simulink model "Haptic feedbck system"  (R2024b)
settings: Solver=ode4  StartTime=0.0  StopTime=inf  FixedStep=0.001  RelTol=1e-3  EnableMultiTasking=on
undefined symbols (not defined in the file): _, cablePTstudyZF, data, date, DiscIntNeverNeededParam, FETau, HIL, i2tTimeLim, iCmd2Volt, iCmdLim, iCmdSat, iCont, iMeasLim, iMeasServoConv, iPeak, iSign, kDposStudyPC, kDstudyZF, kPposStudyPC, kPstudyZF, kS, magnitude, maxTorque, motEncCnts2Rad, motEncSign, motKt, motNegFfTauStudyPC, motPosFfTauStudyPC, motPulleyRad, pulseGuiPeriod, pulseGuiPulseWidth, qc_get_step_size, signals, sprEncCnts2Rad, sprEncSign, tauDzStudyZF, tauJlim, tauMlim, tauNoMvtStudyZF, test_1_robot_torque_, time, tS, Visualization, xJdotLim, xJlimNeg, xJlimPos, xMdotLim, xMlimNeg, xMlimPos
libraries: quarc_library x26, simulink x13, simulink_extras x2
(part 2 of 3)

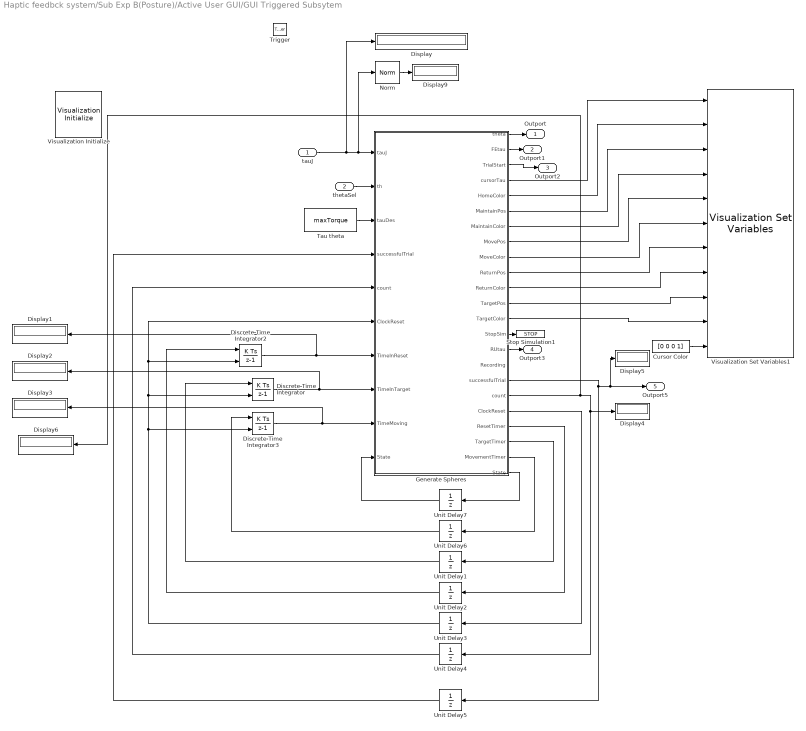
== system Haptic feedbck system/Sub Exp B(Posture)/Active User GUI/GUI Triggered Subsytem ==
  tauJ : Inport
  thetaSel : Inport  Port=2
  Trigger : TriggerPort  VariantControl=(inherit)
  Cursor Color : Constant  Value=[0 0 0 1]  VectorParams1D=off
  Discrete-Time Integrator : DiscreteIntegrator  ExternalReset=rising  SampleTime=-1  OutDataTypeStr=double  ICPrevOutput=DiscIntNeverNeededParam  ICPrevScaledInput=DiscIntNeverNeededParam
  Discrete-Time Integrator2 : DiscreteIntegrator  ExternalReset=rising  SampleTime=-1  OutDataTypeStr=double  ICPrevOutput=DiscIntNeverNeededParam  ICPrevScaledInput=DiscIntNeverNeededParam
  Discrete-Time Integrator3 : DiscreteIntegrator  ExternalReset=rising  SampleTime=-1  OutDataTypeStr=double  ICPrevOutput=DiscIntNeverNeededParam  ICPrevScaledInput=DiscIntNeverNeededParam
  Display{,1..6,9} (8 alike) : Display
  Generate Spheres : MATLAB Function  TreatAsAtomicUnit=on
  Norm : quarc_library/Math Operations/Vectors/Norm
      settings: SourceProductName=QUARC Targets
  Stop Simulation1 : Stop
  Tau theta : Constant  Value=maxTorque  SampleTime=-1
  Unit Delay{1..6} (6 alike) : UnitDelay  SampleTime=-1  HasFrameUpgradeWarning=on
  Unit Delay7 : UnitDelay  InitialCondition=1  SampleTime=-1  StateName=State  HasFrameUpgradeWarning=on
  Visualization Initialize : quarc_library/User Interface/Visualization/Visualization Initialize  object_name=Visualization-1  scene_file=untitled.xml  uri=shmem://%m:1?private=visual  server_send_size=1000000  server_receive_size=1000  derive_from_server=on  client_send_size=1000  client_receive_size=1000000  variables=[ 20 24 34 40 44 50 54 60 64 70 74 ]  initial_values=single([ 0 0 0 1 1 1 1 1 1 1 1 -0.01 0 0 0 0 0 1 0 0 1 0 1 0 1 0 0 0 1 1 1 1 0 0 0 1 1 1 1 ])  open_on_start=on  close_on_stop=off
      settings: AttributesFormatString=%<object_name>  SourceProductName=QUARC Targets
  Visualization Set Variables1 : quarc_library/User Interface/Visualization/Visualization Set Variables  object_name=Visualization-1  offset=[ 11 7 32 35 0 3 25 28 18 21 14 ]  data_type=[ 0 0 0 0 0 0 0 0 0 0 0 ]  length=[ 3 4 3 4 3 4 3 4 3 4 4 ]  sample_time=visualization_get_frame_period  actor_name={'actor.cursor/Position';'actor.home/Diffuse Color';'actor.maintain/Position';'actor.maintain/Diffuse Color';'actor.move/Position';'actor.move/Diffuse Color';'actor.return/Position';'actor.return/Diffuse Color';'actor.target/Position';'actor.target/Diffuse Color';'actor.cursor/Diffuse Color'}
      settings: AttributesFormatString=(%<object_name>)  SourceProductName=QUARC Targets
  Outport : Outport
  Outport1 : Outport  Port=2
  Outport2 : Outport  Port=3
  Outport3 : Outport  Port=4
  Outport5 : Outport  Port=5
  wires:
  thetaSel/1 -> Generate Spheres/2(th)
  Tau theta/1 -> Generate Spheres/3(tauDes)
  tauJ/1 -> Display/1, Norm/1, Generate Spheres/1(tauJ)
  Generate Spheres/19(ClockReset) -> Unit Delay3/1
  Generate Spheres/4(cursorTau) -> Visualization Set Variables1/1
  Generate Spheres/21(TargetTimer) -> Unit Delay1/1
  Unit Delay4/1 -> Generate Spheres/5("count ")
  Generate Spheres/17(successfulTrial) -> Display5/1, Outport5/1, Unit Delay5/1
  Unit Delay5/1 -> Generate Spheres/4("successfulTrial ")
  Unit Delay3/1 -> Generate Spheres/6("ClockReset "), Discrete-Time Integrator2/2, Discrete-Time Integrator/2, Discrete-Time Integrator3/2
  Norm/1 -> Display9/1
  Generate Spheres/20(ResetTimer) -> Unit Delay2/1
  Discrete-Time Integrator3/1 -> Display3/1, Generate Spheres/9(TimeMoving)
  Generate Spheres/22(MovementTimer) -> Unit Delay6/1
  Unit Delay2/1 -> Discrete-Time Integrator2/1
  Discrete-Time Integrator2/1 -> Display1/1, Generate Spheres/7(TimeInReset)
  Unit Delay1/1 -> Discrete-Time Integrator/1
  Unit Delay6/1 -> Discrete-Time Integrator3/1
  Discrete-Time Integrator/1 -> Display2/1, Generate Spheres/8(TimeInTarget)
  Generate Spheres/23(State) -> Unit Delay7/1
  Unit Delay7/1 -> Generate Spheres/10("State ")
  Generate Spheres/5(HomeColor) -> Visualization Set Variables1/2
  Generate Spheres/6(MaintainPos) -> Visualization Set Variables1/3
  Generate Spheres/7(MaintainColor) -> Visualization Set Variables1/4
  Generate Spheres/8(MovePos) -> Visualization Set Variables1/5
  Generate Spheres/9(MoveColor) -> Visualization Set Variables1/6
  Generate Spheres/10(ReturnPos) -> Visualization Set Variables1/7
  Generate Spheres/11(ReturnColor) -> Visualization Set Variables1/8
  Generate Spheres/12(TargetPos) -> Visualization Set Variables1/9
  Generate Spheres/13(TargetColor) -> Visualization Set Variables1/10
  Cursor Color/1 -> Visualization Set Variables1/11
  Generate Spheres/1(theta) -> Outport/1
  Generate Spheres/2(FEtau) -> Outport1/1
  Generate Spheres/3(TrialStart) -> Outport2/1
  Generate Spheres/15(RUtau) -> Outport3/1
  Generate Spheres/14(StopSim) -> Stop Simulation1/1
  Generate Spheres/18(count) -> Display6/1, Display4/1, Unit Delay4/1

== system Haptic feedbck system/Sub Exp B(Posture)/Active UserData Recording/Enabled Subsystem1 ==
  In1 : Inport
  Enable : EnablePort
  To Host File : quarc_library/Sinks/To Host/To Host File  source=Specify via dialog (do not evaluate)  file_name=Main_study_p3_C2_F_R1  variable_name=data  decimation=1  sample_time=-1  file_format=CSV-file  options=Include header only  append=off  final_file_name=Main_study_p3_C2_F_R1.csv  bitrate=2000000
  wires:
  In1/1 -> To Host File/1

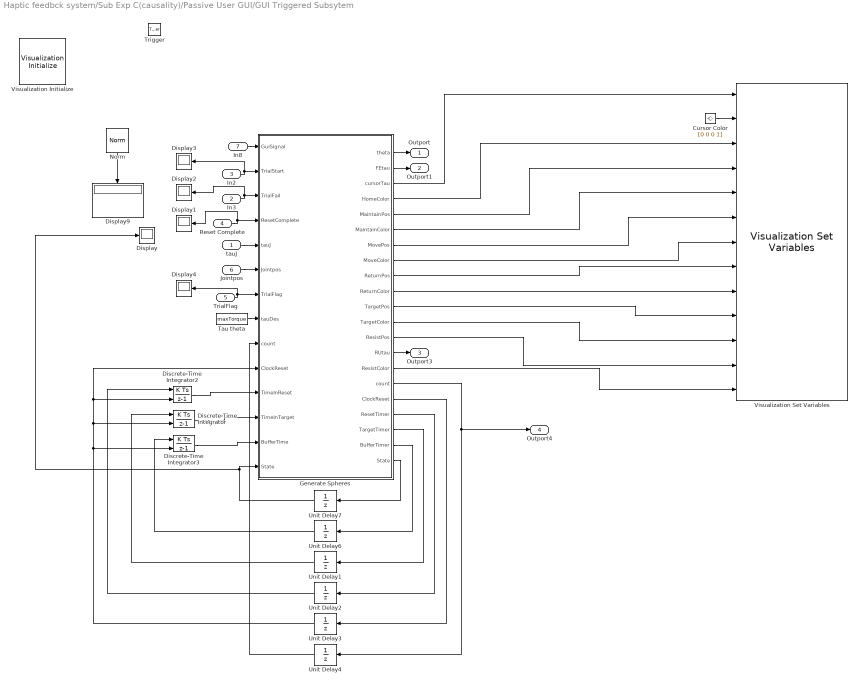
== system Haptic feedbck system/Sub Exp C(causality)/Passive User GUI/GUI Triggered Subsytem ==
  tauJ : Inport
  In3 : Inport  Port=2
  In2 : Inport  Port=3
  Reset Complete : Inport  Port=4
  TrialFlag : Inport  Port=5
  Jointpos : Inport  Port=6
  In8 : Inport  Port=7
  Trigger : TriggerPort  VariantControl=(inherit)
  Cursor Color : Constant  Value=[0 0 0 1]  VectorParams1D=off
  Discrete-Time Integrator : DiscreteIntegrator  ExternalReset=rising  SampleTime=-1  OutDataTypeStr=double  ICPrevOutput=DiscIntNeverNeededParam  ICPrevScaledInput=DiscIntNeverNeededParam
  Discrete-Time Integrator2 : DiscreteIntegrator  ExternalReset=rising  SampleTime=-1  OutDataTypeStr=double  ICPrevOutput=DiscIntNeverNeededParam  ICPrevScaledInput=DiscIntNeverNeededParam
  Discrete-Time Integrator3 : DiscreteIntegrator  ExternalReset=rising  SampleTime=-1  OutDataTypeStr=double  ICPrevOutput=DiscIntNeverNeededParam  ICPrevScaledInput=DiscIntNeverNeededParam
  Display{,1..4,9} (6 alike) : Display
  Generate Spheres : MATLAB Function  TreatAsAtomicUnit=on
  Norm : quarc_library/Math Operations/Vectors/Norm
      settings: SourceProductName=QUARC Targets
  Tau theta : Constant  Value=maxTorque  SampleTime=-1
  Unit Delay{1..4,6} (5 alike) : UnitDelay  SampleTime=-1  HasFrameUpgradeWarning=on
  Unit Delay7 : UnitDelay  SampleTime=-1  StateName=State  HasFrameUpgradeWarning=on
  Visualization Initialize : quarc_library/User Interface/Visualization/Visualization Initialize  object_name=Visualization-1  scene_file=..\exp files\untitled.xml  uri=shmem://%m:1?private=visual  server_send_size=1000000  server_receive_size=1000  derive_from_server=on  client_send_size=1000  client_receive_size=1000000  variables=[ 20 24 30 34 44 50 54 60 64 70 74 80 84 ]  initial_values=single([ -0.01 0 0 0 0 0 1 0 0 0 1 1 1 1 1 1 1 1 0 0 0 1 1 1 1 0 0 0 1 1 1 1 0 0 0 1 1 1 1 0 0 0 1 1 1 1 ])  open_on_start=on  close_on_stop=off
      settings: AttributesFormatString=%<object_name>  SourceProductName=QUARC Targets
  Visualization Set Variables : quarc_library/User Interface/Visualization/Visualization Set Variables  object_name=Visualization-1  offset=[ 0 3 14 25 28 18 21 32 35 7 10 39 42 ]  data_type=[ 0 0 0 0 0 0 0 0 0 0 0 0 0 ]  length=[ 3 4 4 3 4 3 4 3 4 3 4 3 4 ]  sample_time=visualization_get_frame_period  actor_name={'actor.cursor/Position';'actor.cursor/Diffuse Color';'actor.home/Diffuse Color';'actor.maintain/Position';'actor.maintain/Diffuse Color';'actor.move/Position';'actor.move/Diffuse Color';'actor.return/Position';'actor.return/Diffuse Color';'actor.target/Position';'actor.target/Diffuse Color';'actor.resist/Position';'actor.resist/Diffuse Color'}
      settings: AttributesFormatString=(%<object_name>)  SourceProductName=QUARC Targets
  Outport : Outport
  Outport1 : Outport  Port=2
  Outport3 : Outport  Port=3
  Outport4 : Outport  Port=4
  wires:
  Generate Spheres/17(ClockReset) -> Unit Delay3/1
  Generate Spheres/19(TargetTimer) -> Unit Delay1/1
  Unit Delay4/1 -> Generate Spheres/9("count ")
  Unit Delay3/1 -> Generate Spheres/10("ClockReset "), Discrete-Time Integrator2/2, Discrete-Time Integrator/2, Discrete-Time Integrator3/2
  Norm/1 -> Display9/1
  Generate Spheres/18(ResetTimer) -> Unit Delay2/1
  Discrete-Time Integrator3/1 -> Generate Spheres/13(BufferTime)
  Generate Spheres/20(BufferTimer) -> Unit Delay6/1
  Unit Delay2/1 -> Discrete-Time Integrator2/1
  Discrete-Time Integrator2/1 -> Generate Spheres/11(TimeInReset)
  Unit Delay6/1 -> Discrete-Time Integrator3/1
  Discrete-Time Integrator/1 -> Generate Spheres/12(TimeInTarget)
  Generate Spheres/21(State) -> Unit Delay7/1
  Unit Delay7/1 -> Generate Spheres/14("State "), Display/1
  Generate Spheres/1(theta) -> Outport/1
  Generate Spheres/2(FEtau) -> Outport1/1
  Generate Spheres/14(RUtau) -> Outport3/1
  Unit Delay1/1 -> Discrete-Time Integrator/1
  Generate Spheres/3(cursorTau) -> Visualization Set Variables/1
  Cursor Color/1 -> Visualization Set Variables/2
  Generate Spheres/4(HomeColor) -> Visualization Set Variables/3
  Generate Spheres/5(MaintainPos) -> Visualization Set Variables/4
  Generate Spheres/6(MaintainColor) -> Visualization Set Variables/5
  Generate Spheres/7(MovePos) -> Visualization Set Variables/6
  Generate Spheres/8(MoveColor) -> Visualization Set Variables/7
  Generate Spheres/9(ReturnPos) -> Visualization Set Variables/8
  Generate Spheres/10(ReturnColor) -> Visualization Set Variables/9
  Generate Spheres/11(TargetPos) -> Visualization Set Variables/10
  Generate Spheres/12(TargetColor) -> Visualization Set Variables/11
  Generate Spheres/16(count) -> Outport4/1, Unit Delay4/1
  Generate Spheres/13(ResistPos) -> Visualization Set Variables/12
  Generate Spheres/15(ResistColor) -> Visualization Set Variables/13
  tauJ/1 -> Generate Spheres/5(tauJ)
  Jointpos/1 -> Generate Spheres/6(Jointpos)
  TrialFlag/1 -> Display4/1, Generate Spheres/7(TrialFlag)
  Tau theta/1 -> Generate Spheres/8(tauDes)
  Reset Complete/1 -> Generate Spheres/4(ResetComplete), Display1/1
  In3/1 -> Display2/1, Generate Spheres/3(TrialFail)
  In2/1 -> Display3/1, Generate Spheres/2(TrialStart)
  In8/1 -> Generate Spheres/1(GuiSignal)

== system Haptic feedbck system/Sub Exp C(causality)/Passive UserData Recording/Enabled Subsystem1 ==
  In1 : Inport
  Enable : EnablePort
  To Host File : quarc_library/Sinks/To Host/To Host File  source=Specify via dialog (do not evaluate)  file_name=Main_study_p3_C3_R1  variable_name=data  decimation=1  sample_time=-1  file_format=CSV-file  options=Include header only  append=off  final_file_name=Main_study_p3_C3_R1.csv  bitrate=2000000
  wires:
  In1/1 -> To Host File/1

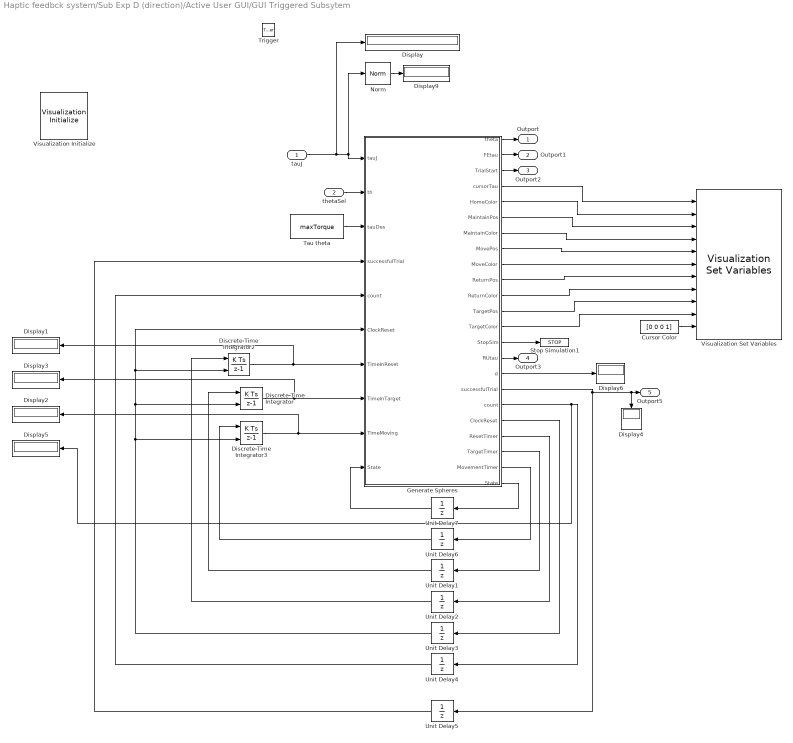
== system Haptic feedbck system/Sub Exp D (direction)/Active User GUI/GUI Triggered Subsytem ==
  tauJ : Inport
  thetaSel : Inport  Port=2
  Trigger : TriggerPort  VariantControl=(inherit)
  Cursor Color : Constant  Value=[0 0 0 1]  VectorParams1D=off
  Discrete-Time Integrator : DiscreteIntegrator  ExternalReset=rising  SampleTime=-1  OutDataTypeStr=double  ICPrevOutput=DiscIntNeverNeededParam  ICPrevScaledInput=DiscIntNeverNeededParam
  Discrete-Time Integrator2 : DiscreteIntegrator  ExternalReset=rising  SampleTime=-1  OutDataTypeStr=double  ICPrevOutput=DiscIntNeverNeededParam  ICPrevScaledInput=DiscIntNeverNeededParam
  Discrete-Time Integrator3 : DiscreteIntegrator  ExternalReset=rising  SampleTime=-1  OutDataTypeStr=double  ICPrevOutput=DiscIntNeverNeededParam  ICPrevScaledInput=DiscIntNeverNeededParam
  Display{,1..6,9} (8 alike) : Display
  Generate Spheres : MATLAB Function  TreatAsAtomicUnit=on
  Norm : quarc_library/Math Operations/Vectors/Norm
      settings: SourceProductName=QUARC Targets
  Stop Simulation1 : Stop
  Tau theta : Constant  Value=maxTorque  SampleTime=-1
  Unit Delay{1..6} (6 alike) : UnitDelay  SampleTime=-1  HasFrameUpgradeWarning=on
  Unit Delay7 : UnitDelay  InitialCondition=1  SampleTime=-1  StateName=State  HasFrameUpgradeWarning=on
  Visualization Initialize : quarc_library/User Interface/Visualization/Visualization Initialize  object_name=Visualization-2  scene_file=untitled.xml  uri=shmem://%m:1?private=visual  server_send_size=1000000  server_receive_size=1000  derive_from_server=on  client_send_size=1000  client_receive_size=1000000  variables=[ 20 24 34 40 44 50 54 60 64 70 74 ]  initial_values=single([ 0 0 0 1 1 1 1 1 1 1 1 -0.01 0 0 0 0 0 1 0 0 1 0 1 0 1 0 0 0 1 1 1 1 0 0 0 1 1 1 1 ])  open_on_start=on  close_on_stop=off
      settings: AttributesFormatString=%<object_name>  SourceProductName=QUARC Targets
  Visualization Set Variables : quarc_library/User Interface/Visualization/Visualization Set Variables  object_name=Visualization-2  offset=[ 11 7 32 35 0 3 25 28 18 21 14 ]  data_type=[ 0 0 0 0 0 0 0 0 0 0 0 ]  length=[ 3 4 3 4 3 4 3 4 3 4 4 ]  sample_time=visualization_get_frame_period  actor_name={'actor.cursor/Position';'actor.home/Diffuse Color';'actor.maintain/Position';'actor.maintain/Diffuse Color';'actor.move/Position';'actor.move/Diffuse Color';'actor.return/Position';'actor.return/Diffuse Color';'actor.target/Position';'actor.target/Diffuse Color';'actor.cursor/Diffuse Color'}
      settings: AttributesFormatString=(%<object_name>)  SourceProductName=QUARC Targets
  Outport : Outport
  Outport1 : Outport  Port=2
  Outport2 : Outport  Port=3
  Outport3 : Outport  Port=4
  Outport5 : Outport  Port=5
  wires:
  thetaSel/1 -> Generate Spheres/2(th)
  Tau theta/1 -> Generate Spheres/3(tauDes)
  tauJ/1 -> Display/1, Norm/1, Generate Spheres/1(tauJ)
  Generate Spheres/19(ClockReset) -> Unit Delay3/1
  Generate Spheres/4(cursorTau) -> Visualization Set Variables/1
  Generate Spheres/21(TargetTimer) -> Unit Delay1/1
  Unit Delay4/1 -> Generate Spheres/5("count ")
  Generate Spheres/17(successfulTrial) -> Display4/1, Outport5/1, Unit Delay5/1
  Unit Delay5/1 -> Generate Spheres/4("successfulTrial ")
  Unit Delay3/1 -> Generate Spheres/6("ClockReset "), Discrete-Time Integrator2/2, Discrete-Time Integrator/2, Discrete-Time Integrator3/2
  Norm/1 -> Display9/1
  Generate Spheres/20(ResetTimer) -> Unit Delay2/1
  Discrete-Time Integrator3/1 -> Display2/1, Generate Spheres/9(TimeMoving)
  Generate Spheres/22(MovementTimer) -> Unit Delay6/1
  Unit Delay2/1 -> Discrete-Time Integrator2/1
  Discrete-Time Integrator2/1 -> Display1/1, Generate Spheres/7(TimeInReset)
  Unit Delay1/1 -> Discrete-Time Integrator/1
  Unit Delay6/1 -> Discrete-Time Integrator3/1
  Discrete-Time Integrator/1 -> Display3/1, Generate Spheres/8(TimeInTarget)
  Generate Spheres/23(State) -> Unit Delay7/1
  Unit Delay7/1 -> Generate Spheres/10("State ")
  Generate Spheres/5(HomeColor) -> Visualization Set Variables/2
  Generate Spheres/6(MaintainPos) -> Visualization Set Variables/3
  Generate Spheres/7(MaintainColor) -> Visualization Set Variables/4
  Generate Spheres/8(MovePos) -> Visualization Set Variables/5
  Generate Spheres/9(MoveColor) -> Visualization Set Variables/6
  Generate Spheres/10(ReturnPos) -> Visualization Set Variables/7
  Generate Spheres/11(ReturnColor) -> Visualization Set Variables/8
  Generate Spheres/12(TargetPos) -> Visualization Set Variables/9
  Generate Spheres/13(TargetColor) -> Visualization Set Variables/10
  Cursor Color/1 -> Visualization Set Variables/11
  Generate Spheres/1(theta) -> Outport/1
  Generate Spheres/2(FEtau) -> Outport1/1
  Generate Spheres/3(TrialStart) -> Outport2/1
  Generate Spheres/15(RUtau) -> Outport3/1
  Generate Spheres/14(StopSim) -> Stop Simulation1/1
  Generate Spheres/18(count) -> Display5/1, Unit Delay4/1
  Generate Spheres/16(d) -> Display6/1

== system Haptic feedbck system/Sub Exp D (direction)/Active UserData Recording/Enabled Subsystem1 ==
  In1 : Inport
  Enable : EnablePort
  To Host File : quarc_library/Sinks/To Host/To Host File  source=Specify via dialog (do not evaluate)  file_name=Main_study_p1_C4_  variable_name=data  decimation=1  sample_time=-1  file_format=CSV-file  options=Include header only  append=off  final_file_name=Main_study_p1_C4_.csv  bitrate=2000000
  wires:
  In1/1 -> To Host File/1

== matlab function Haptic feedbck system/Sub Exp C(causality)/Passive User Control/MATLAB Function ==
  data: tauIn input; tauOut output; cablePT input; tauDz input; tauNoMvt input
function tauOut = fcn(tauIn,cablePT,tauDz,tauNoMvt)
%#codegen
tauOut = zeros(4,1);

tauFE = tauIn(1);
tauRU = tauIn(2);


if tauFE > tauDz(1)
   tauOut(1:2,1) = [cablePT(1) tauFE]';
elseif tauFE < -tauDz(1)
   tauOut(1:2,1) = [-tauFE cablePT(1)]';
else 
  tauOut(1:2,1) = [tauNoMvt(1) tauNoMvt(1)]';
end


if tauRU > tauDz(2)
   tauOut(3:4,1) = [cablePT(2) tauRU]';
elseif tauRU < -tauDz(2)
   tauOut(3:4,1) = [-tauRU cablePT(2)]';
else 
  tauOut(3:4,1) = [tauNoMvt(2) tauNoMvt(2)]';
end

% if tauFE > tauDz(1)
%    tauOut(1:2,1) = [cablePT(1) tauFE-tauDz(1)]';
% elseif tauFE < tauDz(1)
%    tauOut(1:2,1) = [tauDz(1)-tauFE cablePT(1)]';
% else 
%   tauOut(1:2,1) = [tauNoMvt(1) tauNoMvt(1)]';
% end
% 
% 
% if tauRU > tauDz(2)
%    tauOut(3:4,1) = [cablePT(2) tauRU-tauDz(2)]';
% elseif tauRU < tauDz(2)
%    tauOut(3:4,1) = [tauDz(2)-tauRU cablePT(2)]';
% else 
%   tauOut(3:4,1) = [tauNoMvt(2) tauNoMvt(2)]';
% end

== matlab function Haptic feedbck system/Sub Exp D (direction)/Active User GUI/GUI Triggered Subsytem/Generate Spheres ==
  data: theta output; FEtau output; TrialStart output; tauJ input; th input; tauDes input; successfulTrial input; count input; ClockReset input; TimeInReset input; TimeInTarget input; cursorTau output; HomeColor output; MaintainPos output; MaintainColor output; MovePos output; MoveColor output; ReturnPos output; ReturnColor output; TargetPos output; TargetColor output; StopSim output; RUtau output; d output; successfulTrial output; count output; ClockReset output; ResetTimer output; TargetTimer output; TimeMoving input; MovementTimer output; State output; State input
function [theta, FEtau,TrialStart, cursorTau, HomeColor, MaintainPos, MaintainColor, MovePos, MoveColor, ReturnPos, ReturnColor, TargetPos, TargetColor, StopSim, RUtau,d, successfulTrial, count, ClockReset, ResetTimer, TargetTimer, MovementTimer,  State  ] = fcn(tauJ, th, tauDes ...
    , successfulTrial, count, ClockReset,  TimeInReset, TimeInTarget, TimeMoving,  State  )

%%% Extract %%%
FEtau = tauJ(1);
RUtau = tauJ(2);
MaxTau = tauDes;

%%% rep count%%%
reps=3;
nthRep=1;


%%% Target Selection %%%
offset=90*pi/180;

%th= (0:30:150)*pi/180; 

%th= (180:30:330)*pi/180; 


%th= (0:30:330)*pi/180; %[30 120 240 330]
theta_= count+1;
theta= offset-th(theta_);%*pi/180;
NumTargets= length(th);

% %%% Target Pos %%%
 
 TargetPosx= cos(-theta); 
 TargetPosy= sin(-theta); 
 TargetPos =[0 TargetPosy TargetPosx ]'; %target position (coord of center)


%%% Cursor Pos %%%
cursorTauFE = -FEtau/MaxTau(1); % FE cursor tau
cursorTauRU = RUtau/MaxTau(2); % RU cursor tau
cursorTau = [-0.01 cursorTauFE cursorTauRU]'; % Define, - sign in y is so E is positive
%offset= 0.07158;



%Calculations
 dx=TargetPos(2)-cursorTau(2);
 dy=TargetPos(3)-cursorTau(3);
 d= norm([dx dy]); % distance between cursor and target (distance between centers)
 Dc= norm([cursorTau(2) cursorTau(3)]);% distance between cursor and home 
 Dt= norm(TargetPos); % distance between target and home 
 UserTorqueMag= norm(tauJ);
 
 % %%% Color Change %%%  
 MaintainPos= [0 0 0]'; %[-0.2 0 0.2]';
 MovePos= [0 0 0]';
 ReturnPos= [0 0 0]';
 StopSim=0;
Recording=1;

 % text boxes
 MaintainColor= [1 1 1 0]';
 %MaintainPos= [0.2 0 0.2]';
 MoveColor= [0 0 0 0]';
 ReturnColor= [0 0 0 0]';
 
 %sphere colors
 TargetColor=[0 0 0 0]'; 
 HomeColor=[0.85 0 0 0]';

% triggers
 ResetTimer=0;
 TargetTimer=0;
 MovementTimer=0;
 ClockReset=0;

% Durations
ResetDuration = 30;
MovementDuration   = 5;
TrialDuration = 5;
%BetweenReps=10;

 % flags
 CursorInTarget=0;
 TrialStart=0;
 MovementFlag=0;
 
 
 
% state variables
Reset=0;
CursorOutsideTarget = 1;
CursorEnteredTarget = 2;
TrialInProgress = 3;


if isempty(State)
     State=CursorOutsideTarget;
end

    switch State

        case Reset
                if UserTorqueMag<0.15 %&& TimeInReset<ResetDuration
                            TargetTimer =0;
                            ResetTimer=1;
                            MovementTimer=0;
                            MaintainPos= [0.2 0 0.2]';
                            MaintainColor= [1 1 1 1]';
                            ReturnColor= [0 0 0 0]';
                            TargetColor= [0 0.56 0 0]'; 
                            HomeColor= [0.85 0 0 1]'; % home changes to default color
                            
                            % if successfulTrial==1 && UserTorqueMag<0.05
                            %     successfulTrial=0;
                            % end
                            
               else
                            ClockReset=1;
                            MaintainColor= [0 0 0 0]';
                            ReturnColor= [1 1 1 1]';
                            ReturnPos=[0 -0.3 -0.02]';
                            TargetColor = [0 0 0 0]';   % Yellow (reset phase)
                            HomeColor   = [0 0.56 0 1]';      % Green home
                end

        if count ==NumTargets && UserTorqueMag<0.05
            Recording=0;
            StopSim=1;
        end

        if successfulTrial==1 && UserTorqueMag<0.05
           successfulTrial=0;
        end

        if TimeInReset>=ResetDuration
            ClockReset=1;
            State= CursorOutsideTarget;
            ResetTimer=0;
            MovementTimer=1;
            TargetColor=[0 0.56 0 1]';
            HomeColor=[0.15 0.15 0.15 0]';
            ReturnColor= [1 1 1 0]';
            MaintainColor= [1 1 1 0]';
            MoveColor= [1 1 1 1]';
            MovePos=[0 (TargetPos(2)-0.3) (TargetPos(3)-0.02)]';
        end

        case CursorOutsideTarget
            ResetTimer=0;
            MovementTimer=1;
            TargetColor=[0 0.56 0 1]';
            HomeColor=[0.15 0.15 0.15 0]';
            MaintainColor= [1 1 1 0]';
            MoveColor= [1 1 1 1]';
            MovePos=[0 (TargetPos(2)-0.3) (TargetPos(3)-0.02)]';
            
            if TimeMoving >=MovementDuration
                State=Reset;
                ClockReset=1;
                MovementTimer=0;
                ErrorCheck=2;
            end
            
            if  d<=0.15*Dt %cursor inside target sphere
                ClockReset=0;
                MovementTimer=0;
                State= CursorEnteredTarget;
                TargetColor = [0 0.56 0 1]';
                MaintainColor= [1 1 1 0]';
                MoveColor= [1 1 1 1]';
                MovePos=[0 (TargetPos(2)-0.3) (TargetPos(3)-0.02)]';
            end


        case CursorEnteredTarget
            CursorInTarget=1; %flag set
            TargetColor = [0 0.56 0 1]';
            MaintainColor = [0 0 0 0]';
            MoveColor = [1 1 1 1]';
            MovePos = [0 (TargetPos(2)-0.3) (TargetPos(3)-0.02)]';
            MovementTimer=0;

            if d>0.151*Dt
                State=Reset;
                %CursorInTarget = 0;
            end
            
            if d<=0.05*Dt
                State=TrialInProgress;
                TrialStart=1; 
                TargetTimer=1;
            end

        case TrialInProgress
            if d>0.135   % Left target
                ClockReset=1;
                %CursorInTarget = 0;
                TrialStart = 0;
                State = Reset;
                ErrorCheck = 3;
            else
                MovementTimer=0;
                TargetTimer=1;
                TrialStart = 1;
                TargetColor = [0.85 0 0 1]';
                MaintainColor = [1 1 1 1]';
                MoveColor = [0 0 0 0]';
                MaintainPos = [0 (TargetPos(2)-0.3) (TargetPos(3)-0.02)]';
                HomeColor = [0.15 0.15 0.15 0]';
                ClockReset=0;
                
                if TimeInTarget >=TrialDuration
                    count=count+1;
                    State = Reset;
                    successfulTrial = 1;
                    ClockReset=1;
                    TargetTimer=0;
                    TrialStart = 0;
                    
                end
                
            end
    end

end

== matlab function Haptic feedbck system/Sub Exp C(causality)/Passive User GUI/GUI Triggered Subsytem/Generate Spheres ==
  data: GuiSignal input; TrialStart input; TrialFail input; ResetComplete input; theta output; FEtau output; tauJ input; Jointpos input; TrialFlag input; tauDes input; count input; ClockReset input; TimeInReset input; TimeInTarget input; cursorTau output; HomeColor output; MaintainPos output; MaintainColor output; MovePos output; MoveColor output; ReturnPos output; ReturnColor output; TargetPos output; TargetColor output; ResistPos output; RUtau output; ResistColor output; count output; ClockReset output; ResetTimer output; TargetTimer output; BufferTime input; BufferTimer output; State output; State input
function [theta, FEtau, cursorTau, HomeColor, MaintainPos, MaintainColor, MovePos, MoveColor, ReturnPos, ReturnColor, TargetPos, TargetColor,ResistPos, RUtau, ResistColor,count, ClockReset, ResetTimer, TargetTimer, BufferTimer,  State  ] = fcn( GuiSignal, TrialStart, TrialFail, ResetComplete, tauJ, Jointpos, TrialFlag, tauDes, count, ClockReset, TimeInReset, TimeInTarget, BufferTime,  State)

%%% Extract %%%
FEtau = tauJ(1);
RUtau = tauJ(2);
FEpos = Jointpos(1);
RUpos = -Jointpos(2);
MaxTau = tauDes;

%%% rep count%%%
reps=3;

%%% Joint Limits %%%
xJlim = [120 72 70 60]*pi/180;  % [F E U R], [rad]
MaxJointFE = xJlim(1);  % 2.094 rad (120°)
MaxJointRU = xJlim(3);  % 1.222 rad (70°)

%MaxDeflection= [tauDes(1)/kS(1) tauDes(2)/kS(2)];
MaxAngle= 1;

%%% Target Selection %%%
%count=1;
%offset=90*pi/180;
targets= [0 180]*pi/180;
numTargets=length(targets); %length(targets);
theta_= count+1;
theta= targets(theta_);
%TargetDeflection= [tauDes(1)*cos(rot)/kS(1) tauDes(2)*sin(rot)/kS(2)]; %deflection needed to produce TauDes


%%% Cursor Pos %%%
cursorTauFE = FEtau/MaxTau(1); % FE cursor tau
cursorTauRU = RUtau/MaxTau(2); % RU cursor tau
cursorTau = [-0.01 FEpos/MaxAngle RUpos/MaxAngle]'; % Define, - sign in y is so E is positive
%offset= 0.07158;

% %%% Target Pos %%%
 TargetPosx= cos(theta); 
 TargetPosy= -sin(theta); 
 TargetPos =[0 0 0]'; % [0 0 0]' [0 TargetPosy TargetPosx ]' target position (coord of center)
 

%Calculations
dx=TargetPos(2)-cursorTau(2);
dy=TargetPos(3)-cursorTau(3);
d= norm([dx dy]); % distance between cursor and target (distance between centers)
Dc= norm([cursorTau(2) cursorTau(3)]);% distance between cursor and home
Dt= norm(TargetPos); % distance between target and home
UserTorqueMag= abs(tauJ(1));

 % text boxes
 MaintainPos= [0 0 0]'; %[-0.2 0 0.2]';
 MaintainColor= [1 1 1 0]';

 MovePos= [0 0 0]';
 MoveColor= [0 0 0 0]';

 ReturnPos= [0 0 0]';
 ReturnColor= [0 0 0 0]';

 ResistPos= [0.2 0 0.2]';
 ResistColor= [0 0 0 0]';

 %sphere colors
 TargetColor=[0 0 0 0]'; 
 HomeColor=[0.85 0 0 0]';

% timers
 ResetTimer=0;
 TargetTimer=0;
 BufferTimer=0;
 ClockReset=0;

% Durations
ResetDuration = 5;
BufferDuration   = 2;
TrialDuration = 5;

% 

% state variables
Reset=0;
TrialInProgress = 1;

% if isempty(State)
%      State=Reset;
% end

State = GuiSignal;

    switch State
        
        case 0   % RESET
        
        if Dc < 0.03
            MaintainPos = [0.2 0 0.2]';
            MaintainColor = [1 1 1 1]';
            HomeColor = [0.85 0 0 1]';
        else
            ReturnColor = [1 1 1 1]';
            ReturnPos = [0 -0.3 -0.02]';
            HomeColor = [0 0.56 0 1]';
        end
        
        TargetColor = [0 0 0 0]';
        ResistColor = [0 0 0 0]';


    case 1   % READY
        
        TargetColor = [0.85 0 0 1]';
        HomeColor = [0.15 0.15 0.15 0]';
        ResistColor = [1 1 1 1]';
        ResistPos = [0.4 0 0.4]';


    case 2   % ACTIVE TRIAL
        
        TargetColor = [0.85 0 0 1]';
        ResistColor = [1 1 1 1]';
        ResistPos = [0.4 0 0.4]';
        HomeColor = [0.15 0.15 0.15 0]';


    case 3   % SUCCESS
        
        ReturnColor = [1 1 1 1]';
        ReturnPos = [0 -0.3 -0.02]';
        MaintainColor = [1 1 1 0]';
        TargetColor = [0 0 0 0]';
        HomeColor = [0 0.56 0 1]';


    case 4   % FAIL

        ReturnColor = [1 1 1 1]';
        TargetColor = [0 0 0 0]';
        HomeColor = [0 0.56 0 1]';

      
    end
      
end

== matlab function Haptic feedbck system/Sub Exp D (direction)/Active User Control /MATLAB Function ==
  data: tauIn input; tauOut output; tauPosFF input; tauNegFF input; desAngMag input
function tauOut = fcn(tauIn,tauPosFF,tauNegFF,desAngMag)
%#codegen
tauOut = zeros(4,1);

tauFE = tauIn(1);
tauRU = tauIn(2);
tauPosFFfe = tauPosFF;
tauPosFFru = tauPosFF;

if desAngMag == 0
   tauPosFFfe = 0.1;
   tauPosFFru = 0.1;
end

if tauFE > 0
   tauOut(1:2,1) = [tauNegFF tauFE+tauPosFFfe]';
elseif tauFE < 0
   tauOut(1:2,1) = [tauPosFFfe-tauFE tauNegFF]';
else 
  tauOut(1:2,1) = [0 0]';
end


if tauRU > 0
   tauOut(3:4,1) = [tauNegFF tauRU+tauPosFFru]';
elseif tauRU < 0
   tauOut(3:4,1) = [tauPosFFru-tauRU tauNegFF]';
else 
  tauOut(3:4,1) = [0 0]';
end

== matlab function Haptic feedbck system/Sub Exp B(Posture)/Active User Control /MATLAB Function ==
  data: tauIn input; tauOut output; tauPosFF input; tauNegFF input; desAngMag input
function tauOut = fcn(tauIn,tauPosFF,tauNegFF,desAngMag)
%#codegen
tauOut = zeros(4,1);

tauFE = tauIn(1);
tauRU = tauIn(2);
tauPosFFfe = tauPosFF;
tauPosFFru = tauPosFF;

if desAngMag == 0
   tauPosFFfe = 0.1;
   tauPosFFru = 0.1;
end

if tauFE > 0
   tauOut(1:2,1) = [tauNegFF tauFE+tauPosFFfe]';
elseif tauFE < 0
   tauOut(1:2,1) = [tauPosFFfe-tauFE tauNegFF]';
else 
  tauOut(1:2,1) = [0 0]';
end


if tauRU > 0
   tauOut(3:4,1) = [tauNegFF tauRU+tauPosFFru]';
elseif tauRU < 0
   tauOut(3:4,1) = [tauPosFFru-tauRU tauNegFF]';
else 
  tauOut(3:4,1) = [0 0]';
end

== matlab function Haptic feedbck system/Sub Exp C(causality)/Passive User Control/MATLAB Function1 ==
  settings: updateMethod=DISCRETE  sampleTime=0.001
  data: GuiSignal output; ResetComplete output; ForceLatch output; TrialStart output; TrialComplete output; ErrorCheck output; StopSim output; TauDes output; ClockReset output; BufferTimer output; TrialDurationTimer output; ResetTimer output; RampTimer output; counter output; Jointpos input; maxTorque input; tauJ input; ClockReset input; BufferTime input; TrialTime input; ResetTime input; RampTime input; counter input; state input; state output
function [GuiSignal, ResetComplete, ForceLatch, TrialStart, TrialComplete, ErrorCheck, StopSim,  TauDes, ClockReset, BufferTimer,TrialDurationTimer, ResetTimer, RampTimer, counter, state] = fcn(Jointpos, maxTorque, tauJ, ClockReset,BufferTime, TrialTime, ResetTime, RampTime, counter, state)

%initialization
StopSim= 0;
ResetTimer = 0;
RampTimer = 0;
TrialDurationTimer=0;
BufferTimer=0;
TauDes   = [0 0]; %force applied by robot
UserTau=0; % force applied by user
TrialComplete=0;
%ForceLatch=0;
%ForceMagnitude = 0;

%direction sequence
directions=  [0 180 0 180 0 180]*pi/180;%[0 180][0 180 0 180
numDirections= length(directions);


%current direction
theta_= counter+1;
theta = directions(theta_);
u_dir = [cos(theta) sin(theta)]; %force direction

%reference points
FEpos = Jointpos(1);
RUpos = Jointpos(2);
CursorDist= norm([FEpos RUpos]);


% Durations
ResetDuration = 30;
TrialDuration = 5;
BufferDuration=2;
StopSim=0;


% flags
 TrialStart=0;
 ResetComplete=0;
 ErrorCheck=0;
 ForceLatch=0;

%applied user force threshold
UserTauThresh= maxTorque(1);
UserTauThreshU= 1.25*maxTorque(1);
UserTauThreshL= 0.75*maxTorque(1);
UserTau = norm(tauJ);
 
% state variables
Reset=0;
RampUp = 1; 
ForceLock=2;
TrialPeriod=3;
RampDown=4;

if isempty(state)
    state = RampUp;
end

persistent TauPrev ThresholdExceeded RampDownStartForce ForceMagnitude LatchedState

if isempty(LatchedState)
    LatchedState = 1;
end

if isempty(ForceMagnitude)
    ForceMagnitude = 0;
end


if isempty(TauPrev)
    TauPrev = [0 0];
end


if isempty(ThresholdExceeded)
    ThresholdExceeded = false;
end


if isempty(RampDownStartForce)
    RampDownStartForce = [0 0];
end

switch state

    case Reset
        %  TrialLock=0;
            UserTau = 0;
            TauDes = [0 0];
            RampTimer = 0;
            TrialDurationTimer = 0;
            ThresholdExceeded = false;
            TauPrev = [0 0];
            RampDownStartForce = [0 0];

        if  CursorDist<0.03 && ResetTime<=ResetDuration %&& ResetComplete~=1
                ResetTimer = 1;
                ClockReset=0;

        elseif CursorDist> 0.08 && ResetTime<=ResetDuration %ResetTime< ResetDuration %&& MovementFlag~=1 CursorDist> 0.02
                ResetTimer = 0;
                ClockReset=1;

        end

        if counter ==numDirections && CursorDist<0.03
                    StopSim=1;
       end 

        if ResetTime > ResetDuration  %ResetTime > ResetDuration %&& ResetComplete==1 
            state= RampUp;
            ResetComplete=1;
            ClockReset=1;
            ResetTimer=0;
        end
    
    case RampUp
        ClockReset=0;
        RampTimer = 1;
        ResetComplete=0;

        %%Force Ramp
        
        ForceRate= 0.5; %ramp for force applied by robot (Nm/s)
        if ~ThresholdExceeded 
            ForceMagnitude= ForceRate*RampTime; 
            TauDes = ForceMagnitude * u_dir;
        % else 
        %     RampTimer = 0; 
        %     TauDes = TauPrev; %Hold the force constant once resistance is detected 
        end
         

        % User exceeds torque threshold
        if UserTau > UserTauThresh && ~ThresholdExceeded %UserTau >= UserTauThresh ForceLatch == 1
            ForceLatch=1;
            RampTimer = 0;
            ClockReset = 1;     % reset timer for hold
            ThresholdExceeded = true;
            TauPrev = TauDes;   % lock force
            state = ForceLock;
        end

         if RampTime>=15
            state = RampDown;
            RampDownStartForce = TauDes; 
        end
    
    case ForceLock
        
        ClockReset=0;
        TauDes = TauPrev;
        ForceLatch=1;
        % BufferTimer=1;

        % Clock to track total for ForceLock
        RampTimer = 1;

         if ThresholdExceeded && UserTau > UserTauThreshL %&& TrialStart==1 %&& UserTau < 1.15*maxTorque(1) && UserTau > 0.85*maxTorque(1)
             %state= TrialPeriod;
              BufferTimer=1;
         elseif UserTau > UserTauThreshU 
              state = RampDown;
              RampDownStartForce = TauPrev;    
         else
             BufferTimer=0;
             ClockReset=1;
         end

         if BufferTime>=BufferDuration
             state= TrialPeriod;
             ForceLatch=0;
             BufferTimer=0;
             ClockReset=1;
         end

         if RampTime>=4
            state = RampDown;
            RampDownStartForce = TauPrev; 
         end

     % Trial
    case TrialPeriod
         
         TauDes = TauPrev;
         ClockReset = 0; 

        if  UserTau < UserTauThreshU && UserTau > UserTauThreshL % trial complete ThresholdExceeded && 
                TrialDurationTimer = 1;
                TrialStart=1;

        elseif  UserTau > UserTauThreshU || UserTau < UserTauThreshL
                TrialDurationTimer=0;
                TrialStart=0;
                ErrorCheck=1;
                ClockReset = 1;
                RampDownStartForce = TauPrev; 
                state = RampDown;     
        end

        if TrialTime>=TrialDuration
            state = RampDown;
            RampDownStartForce = TauPrev; 
            counter=counter+1;
            TrialStart=0;
            TrialComplete=1;
        end



    case RampDown
        % Smooth ramp down to zero
        ErrorCheck=0;
        ClockReset = 0; 
        TrialComplete=0;
        ResetTimer = 0;
        RampDownDuration = 2;

        if RampTime < RampDownDuration
            % Linear ramp down
            s = 1 - (RampTime / RampDownDuration);
            TauDes = s * RampDownStartForce;
            RampTimer = 1;
        else
            % Ramp complete, go to reset
            TauDes = [0 0];
            state = Reset;
            ClockReset = 1;
            RampTimer = 0;
        end
        TrialDurationTimer = 0;

end

switch LatchedState

    case 0  % Reset
        if ResetComplete == 1
            LatchedState = 1;
        end

    case 1  % Ready
        if ForceLatch==1
            LatchedState = 2;
        end

    case 2  % Active
        if TrialStart==1
            LatchedState = 2;
        elseif  ErrorCheck== 1
            LatchedState = 0;
       elseif TrialComplete == 1         
            LatchedState = 0;
        end

    case 3  % Success
        if state == RampDown
            LatchedState = 3;
        end

    case 4  % Fail
        if ErrorCheck== 1
            LatchedState = 0;
        end

end

% if ThresholdExceeded
%     TauDes = TauPrev;
% end

GuiSignal = LatchedState;

end

== matlab function Haptic feedbck system/Sub Exp B(Posture)/Active User GUI/GUI Triggered Subsytem/Generate Spheres ==
  data: theta output; FEtau output; TrialStart output; tauJ input; th input; tauDes input; successfulTrial input; count input; ClockReset input; TimeInReset input; TimeInTarget input; cursorTau output; HomeColor output; MaintainPos output; MaintainColor output; MovePos output; MoveColor output; ReturnPos output; ReturnColor output; TargetPos output; TargetColor output; StopSim output; RUtau output; Recording output; successfulTrial output; count output; ClockReset output; ResetTimer output; TargetTimer output; TimeMoving input; MovementTimer output; State output; State input
function [theta, FEtau,TrialStart, cursorTau, HomeColor, MaintainPos, MaintainColor, MovePos, MoveColor, ReturnPos, ReturnColor, TargetPos, TargetColor, StopSim, RUtau, Recording, successfulTrial, count, ClockReset, ResetTimer, TargetTimer, MovementTimer,  State  ] = fcn(tauJ, th, tauDes ...
    , successfulTrial, count,ClockReset,  TimeInReset, TimeInTarget, TimeMoving,  State  )

%%% Extract %%%
FEtau = tauJ(1);
RUtau = tauJ(2);
MaxTau = tauDes;

%%% rep count%%%
reps=3;
nthRep=1;


%%% Target Selection %%%
offset=90*pi/180;
%th= (0:30:330);
theta_= count+1;
theta= offset-th(theta_);%*pi/180;
NumTargets= length(th);

% %%% Target Pos %%%
 
 TargetPosx= cos(-theta); 
 TargetPosy= sin(-theta); 
 TargetPos =[0 TargetPosy TargetPosx ]'; %target position (coord of center)


%%% Cursor Pos %%%
cursorTauFE = -FEtau/MaxTau(1); % FE cursor tau
cursorTauRU = RUtau/MaxTau(2); % RU cursor tau
cursorTau = [-0.01 cursorTauFE cursorTauRU]'; % Define, - sign in y is so E is positive
%offset= 0.07158;



%Calculations
 dx=TargetPos(2)-cursorTau(2);
 dy=TargetPos(3)-cursorTau(3);
 d= norm([dx dy]); % distance between cursor and target (distance between centers)
 Dc= norm([cursorTau(2) cursorTau(3)]);% distance between cursor and home 
 Dt= norm(TargetPos); % distance between target and home 
 UserTorqueMag= norm(tauJ);
 
 % %%% Color Change %%%  
 MaintainPos= [0 0 0]'; %[-0.2 0 0.2]';
 MovePos= [0 0 0]';
 ReturnPos= [0 0 0]';
 StopSim=0;
 Recording=1;

 % text boxes
 MaintainColor= [1 1 1 0]';
 %MaintainPos= [0.2 0 0.2]';
 MoveColor= [0 0 0 0]';
 ReturnColor= [0 0 0 0]';
 
 %sphere colors
 TargetColor=[0 0 0 0]'; 
 HomeColor=[0.85 0 0 0]';

% triggers
 ResetTimer=0;
 TargetTimer=0;
 MovementTimer=0;
 ClockReset=0;

% Durations
ResetDuration = 30;
MovementDuration   = 5;
TrialDuration = 5;
BetweenReps=10;

 % flags
 CursorInTarget=0;
 TrialStart=0;
 MovementFlag=0;
 
 
 
% state variables
Reset=0;
CursorOutsideTarget = 1;
CursorEnteredTarget = 2;
TrialInProgress = 3;


if isempty(State)
     State=CursorOutsideTarget;
end

    switch State

        case Reset
                 if UserTorqueMag<0.15 %&& TimeInReset<ResetDuration
                            TargetTimer =0;
                            ResetTimer=1;
                            MovementTimer=0;
                            MaintainPos= [0.2 0 0.2]';
                            MaintainColor= [1 1 1 1]';
                            ReturnColor= [0 0 0 0]';
                            TargetColor= [0 0.56 0 0]'; 
                            HomeColor= [0.85 0 0 1]'; % home changes to default color
                            
                            % if successfulTrial==1 && UserTorqueMag<0.05
                            %     successfulTrial=0;
                            % end
                            
               else
                            ClockReset=1;
                            MaintainColor= [0 0 0 0]';
                            ReturnColor= [1 1 1 1]';
                            ReturnPos=[0 -0.3 -0.02]';
                            TargetColor = [0 0 0 0]';   % Yellow (reset phase)
                            HomeColor   = [0 0.56 0 1]';      % Green home
                end

        if count ==NumTargets && UserTorqueMag<0.05
            Recording=0;
            StopSim=1;
        end

        if successfulTrial==1 && UserTorqueMag<0.05
           successfulTrial=0;
        end

        if TimeInReset>=ResetDuration
            ClockReset=1;
            State= CursorOutsideTarget;
            ResetTimer=0;
            MovementTimer=1;
            TargetColor=[0 0.56 0 1]';
            HomeColor=[0.15 0.15 0.15 0]';
            ReturnColor= [1 1 1 0]';
            MaintainColor= [1 1 1 0]';
            MoveColor= [1 1 1 1]';
            MovePos=[0 (TargetPos(2)-0.3) (TargetPos(3)-0.02)]';
        end

        case CursorOutsideTarget
            ResetTimer=0;
            MovementTimer=1;
            TargetColor=[0 0.56 0 1]';
            HomeColor=[0.15 0.15 0.15 0]';
            MaintainColor= [1 1 1 0]';
            MoveColor= [1 1 1 1]';
            MovePos=[0 (TargetPos(2)-0.3) (TargetPos(3)-0.02)]';
            
            % if TimeMoving >=MovementDuration
            %     State=Reset;
            %     ClockReset=1;
            %     MovementTimer=0;
            %     ErrorCheck=2;
            % end
            
            if  d<=0.15*Dt %cursor inside target sphere
                ClockReset=0;
                MovementTimer=0;
                State= CursorEnteredTarget;
                TargetColor = [0 0.56 0 1]';
                MaintainColor= [1 1 1 0]';
                MoveColor= [1 1 1 1]';
                MovePos=[0 (TargetPos(2)-0.3) (TargetPos(3)-0.02)]';
            end


        case CursorEnteredTarget
            CursorInTarget=1; %flag set
            TargetColor = [0 0.56 0 1]';
            MaintainColor = [0 0 0 0]';
            MoveColor = [1 1 1 1]';
            MovePos = [0 (TargetPos(2)-0.3) (TargetPos(3)-0.02)]';
            MovementTimer=0;

            if d>0.151*Dt
                State=Reset;
                %CursorInTarget = 0;
            end
            
            if d<=0.05*Dt
                State=TrialInProgress;
                TrialStart=1; 
                TargetTimer=1;
            end

        case TrialInProgress
            if d>0.135   % Left target
                ClockReset=1;
                CursorInTarget = 0;
                TrialStart = 0;
                State = Reset;
                ErrorCheck = 3;
            else
                MovementTimer=0;
                TargetTimer=1;
                TrialStart = 1;
                TargetColor = [0.85 0 0 1]';
                MaintainColor = [1 1 1 1]';
                MoveColor = [0 0 0 0]';
                MaintainPos = [0 (TargetPos(2)-0.3) (TargetPos(3)-0.02)]';
                HomeColor = [0.15 0.15 0.15 0]';
                ClockReset=0;
                
                if TimeInTarget >=TrialDuration
                    count=count+1;
                    State = Reset;
                    successfulTrial = 1;
                    ClockReset=1;
                    TargetTimer=0;
                    TrialStart = 0;
                    
                end
            end
    end

end

== matlab function Haptic feedbck system/Sub Exp A(Baseline)/Active User Control /MATLAB Function ==
  data: tauIn input; tauOut output; tauPosFF input; tauNegFF input; desAngMag input
function tauOut = fcn(tauIn,tauPosFF,tauNegFF,desAngMag)
%#codegen
tauOut = zeros(4,1);

tauFE = tauIn(1);
tauRU = tauIn(2);
tauPosFFfe = tauPosFF;
tauPosFFru = tauPosFF;

if desAngMag == 0
   tauPosFFfe = 0.1;
   tauPosFFru = 0.1;
end

if tauFE > 0
   tauOut(1:2,1) = [tauNegFF tauFE+tauPosFFfe]';
elseif tauFE < 0
   tauOut(1:2,1) = [tauPosFFfe-tauFE tauNegFF]';
else 
  tauOut(1:2,1) = [0 0]';
end


if tauRU > 0
   tauOut(3:4,1) = [tauNegFF tauRU+tauPosFFru]';
elseif tauRU < 0
   tauOut(3:4,1) = [tauPosFFru-tauRU tauNegFF]';
else 
  tauOut(3:4,1) = [0 0]';
end

== matlab function Haptic feedbck system/Pos Ramp/MATLAB Function ==
  data: tauIn input; tauOut output; tauPosFF input; tauNegFF input; desAngMag input
function tauOut = fcn(tauIn,tauPosFF,tauNegFF,desAngMag)
%#codegen
tauOut = zeros(4,1);

tauFE = tauIn(1);
tauRU = tauIn(2);
tauPosFFfe = tauPosFF;
tauPosFFru = tauPosFF;

if desAngMag == 0
   tauPosFFfe = 0.1;
   tauPosFFru = 0.1;
end

if tauFE > 0
   tauOut(1:2,1) = [tauNegFF tauFE+tauPosFFfe]';
elseif tauFE < 0
   tauOut(1:2,1) = [tauPosFFfe-tauFE tauNegFF]';
else 
  tauOut(1:2,1) = [0 0]';
end


if tauRU > 0
   tauOut(3:4,1) = [tauNegFF tauRU+tauPosFFru]';
elseif tauRU < 0
   tauOut(3:4,1) = [tauPosFFru-tauRU tauNegFF]';
else 
  tauOut(3:4,1) = [0 0]';
end

== matlab function Haptic feedbck system/Pos Ramp/MATLAB Function1 ==
  data: t input; desired_pos output; start_pos input; target_pos input; duration input
function desired_pos  = trajectory_generator(t, start_pos, target_pos, duration)
    % TRAJECTORY_GENERATOR Generates smooth 5th order polynomial trajectory
    %
    % Inputs:
    %   t          - Current time (scalar)
    %   start_pos  - Starting position (vector, e.g., [0; 0])
    %   target_pos - Target position (vector, e.g., [30; 0])
    %   duration   - Duration of trajectory (scalar, e.g., 3.0)
    %
    % Outputs:
    %   desired_pos - Desired position at time t
    %   desired_vel - Desired velocity at time t
    %   desired_acc - Desired acceleration at time t
    
    % Ensure column vectors
    start_pos = start_pos(:);
    target_pos = target_pos(:);
    
    % Compute displacement
    delta = target_pos - start_pos;
    
    % Normalized time
    if t <= 0
        tau = 0;
    elseif t >= duration
        tau = 1;
    else
        tau = t / duration;
    end
    
    % 5th order polynomial and derivatives
    % s(tau) = 10*tau^3 - 15*tau^4 + 6*tau^5
    s = 10*tau^3 - 15*tau^4 + 6*tau^5;
    
    % ds/dtau = 30*tau^2 - 60*tau^3 + 30*tau^4
    if t > 0 && t < duration
        ds_dtau = 30*tau^2 - 60*tau^3 + 30*tau^4;
        ds_dt = ds_dtau / duration;
    else
        ds_dt = 0;
    end
    
    % d2s/dtau2 = 60*tau - 180*tau^2 + 120*tau^3
    if t > 0 && t < duration
        d2s_dtau2 = 60*tau - 180*tau^2 + 120*tau^3;
        d2s_dt2 = d2s_dtau2 / (duration^2);
    else
        d2s_dt2 = 0;
    end
    
    % Compute outputs
    desired_pos = start_pos + s * delta;
    desired_vel = ds_dt * delta;
    desired_acc = d2s_dt2 * delta;
end
